simulink model "Iteration3_Transformer_classAmplifier"  (R2015a)
settings: Solver=ode23t  StartTime=0.0  StopTime=1e-2  RelTol=1e-3
libraries: fl_lib x9, elec_lib x9, nesl_utility x6
settings Model: Creator=saifur  LastModifiedBy=saifur
settings DebuggingCC: UnconnectedInputMsg=none  UnconnectedOutputMsg=none  UnconnectedLineMsg=none

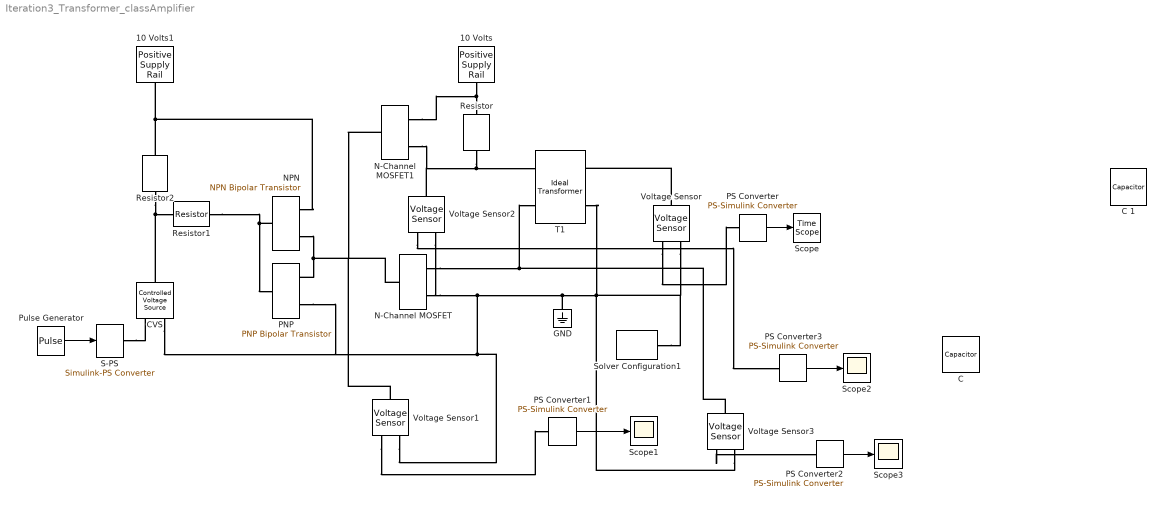
== system Iteration3_Transformer_classAmplifier ==
  " C " : fl_lib/Electrical/Electrical Elements/Capacitor  c=1e-6 F  r=1e-6 Ohm  g=0 1/Ohm  i_specify=off  i_priority=High  i=0 A  v_specify=off  v_priority=High  v=0 V  vc_specify=off  vc_priority=High  vc=0 V
  " C 1" : fl_lib/Electrical/Electrical Elements/Capacitor  c=4700e-6 F  r=1e-6 Ohm  g=0 1/Ohm  i_specify=off  i_priority=High  i=0 A  v_specify=off  v_priority=High  v=0 V  vc_specify=off  vc_priority=High  vc=0 V
  10 Volts : elec_lib/Sources/Positive Supply Rail  v0=5 V
  10 Volts1 : elec_lib/Sources/Positive Supply Rail  v0=5 V
  CVS : fl_lib/Electrical/Electrical Sources/Controlled Voltage Source
  GND : fl_lib/Electrical/Electrical Elements/Electrical Reference
  N-Channel MOSFET : elec_lib/Semiconductor Devices/N-Channel MOSFET  parameterization=1  prmDatasheet=1  prmEquCoeff=1  Beta=5 A/V^2  Rds=0.025 Ohm  Id=6 A  Vgs=10 V  Vth=1.7 V  lam=0 1/V  Tmeas=25 C  RS=1e-4 Ohm  RD=0.01 Ohm  C_param=1  C_GS=270 pF  C_GD=80 pF  C_iss=350 pF  C_rss=80 pF  C_oss=0 pF  C_GS_vec=[ 270 300 290 280 295 255 ] pF  C_GD_vec=[ 450 400 300 190 95 55 ] pF  C_iss_vec=[ 720 700 590 470 390 310 ] pF  C_rss_vec=[ 450 400 300 190 95 55 ] pF  C_oss_vec=[ 900 810 690 420 270 170 ] pF  C_Vds_vec=[ 0.1 0.3 1 3 10 30 ] V  charge_linearity_param=1  C_OX=200 pF  V_C_OX=-0.5 V  dVth_dT=-6 mV/K  Rds_T2=0.037 Ohm  Tmeas2=125 C  BEXDatasheet=-1.5  BEXEquCoeff=-1.5  TdeviceDatasheet=25 C  TdeviceEquCoeff=25 C  Rth=[ 0 10 ] K/W  thermal_mass_parameterization=1  thermal_mass=[ 0 1 ] J/K  thermal_time_constant=[ 0 10 ] s  thermal_mass_initial_temperatures=[ 25 25 ] C
  N-Channel MOSFET1 : elec_lib/Semiconductor Devices/N-Channel MOSFET  parameterization=1  prmDatasheet=1  prmEquCoeff=1  Beta=5 A/V^2  Rds=0.025 Ohm  Id=6 A  Vgs=10 V  Vth=1.7 V  lam=0 1/V  Tmeas=25 C  RS=1e-4 Ohm  RD=0.01 Ohm  C_param=1  C_GS=270 pF  C_GD=80 pF  C_iss=350 pF  C_rss=80 pF  C_oss=0 pF  C_GS_vec=[ 270 300 290 280 295 255 ] pF  C_GD_vec=[ 450 400 300 190 95 55 ] pF  C_iss_vec=[ 720 700 590 470 390 310 ] pF  C_rss_vec=[ 450 400 300 190 95 55 ] pF  C_oss_vec=[ 900 810 690 420 270 170 ] pF  C_Vds_vec=[ 0.1 0.3 1 3 10 30 ] V  charge_linearity_param=1  C_OX=200 pF  V_C_OX=-0.5 V  dVth_dT=-6 mV/K  Rds_T2=0.037 Ohm  Tmeas2=125 C  BEXDatasheet=-1.5  BEXEquCoeff=-1.5  TdeviceDatasheet=25 C  TdeviceEquCoeff=25 C  Rth=[ 0 10 ] K/W  thermal_mass_parameterization=1  thermal_mass=[ 0 1 ] J/K  thermal_time_constant=[ 0 10 ] s  thermal_mass_initial_temperatures=[ 25 25 ] C
  "NPN " : elec_lib/Semiconductor Devices/NPN Bipolar Transistor  parameterization=1  prmDatasheet=1  prmEquCoeff=1  BF=100  IS=1e-14 A  ec=1  VAF=200 V  hfe=100  hoe=5e-5 1/Ohm  Ic_h=1 mA  Vce_h=5 V  V1=0.55 V  I1=0.5 mA  BR=1  Tmeas=25 C  RC=0.01 Ohm  RE=1e-4 Ohm  RB=1 Ohm  C_BC=5 pF  C_BE=5 pF  TF=0 us  TR=0 us  hfe_T2=125  XTB=0  V1_T2=0.45 V  I1_T2=0.5 mA  Tmeas2=125 C  EG=1.11 eV  XTI=3  TdeviceDatasheet=25 C  TdeviceEquCoeff=25 C  Rth=[ 0 10 ] K/W  thermal_mass_parameterization=1  thermal_mass=[ 0 1 ] J/K  thermal_time_constant=[ 0 10 ] s  thermal_mass_initial_temperatures=[ 25 25 ] C
  "PNP " : elec_lib/Semiconductor Devices/PNP Bipolar Transistor  parameterization=1  prmDatasheet=1  prmEquCoeff=1  BF=100  IS=1e-14 A  ec=1  VAF=200 V  hfe=100  hoe=5e-5 1/Ohm  Ic_h=-1 mA  Vce_h=-5 V  V1=-0.55 V  I1=-0.5 mA  BR=1  Tmeas=25 C  RC=0.01 Ohm  RE=1e-4 Ohm  RB=1 Ohm  C_BC=5 pF  C_BE=5 pF  TF=0 us  TR=0 us  hfe_T2=125  XTB=0  V1_T2=-0.45 V  I1_T2=-0.5 mA  Tmeas2=125 C  EG=1.11 eV  XTI=3  TdeviceDatasheet=25 C  TdeviceEquCoeff=25 C  Rth=[ 0 10 ] K/W  thermal_mass_parameterization=1  thermal_mass=[ 0 1 ] J/K  thermal_time_constant=[ 0 10 ] s  thermal_mass_initial_temperatures=[ 25 25 ] C
  PS Converter{,1..3} (4 alike) : nesl_utility/PS-Simulink Converter  PhysicalDomain=network_engine_domain  SubClassName=ps_output  LeftPortType=input  RightPortType=output  PseudoPeriodic=off  Frequencies=[]  Unit=1  AffineConversion=off
  Pulse Generator : DiscretePulseGenerator  PulseType=Time based  Amplitude=5  Period=0.000005  PulseWidth=50
  Resistor : elec_lib/Passive Devices/Resistor  R=100 kOhm  noise_mode=0  Tdevice=25 C  sample_time=0.001 s  repeatability=1  auto_seed=696567710  user_seed=0
  Resistor1 : elec_lib/Passive Devices/Resistor  R=10 Ohm  noise_mode=0  Tdevice=25 C  sample_time=0.001 s  repeatability=1  auto_seed=2103192391  user_seed=0
  Resistor2 : elec_lib/Passive Devices/Resistor  R=100 Ohm  noise_mode=0  Tdevice=25 C  sample_time=0.001 s  repeatability=1  auto_seed=1458113108  user_seed=0
  "S-PS " : nesl_utility/Simulink-PS Converter  PhysicalDomain=network_engine_domain  SubClassName=ps_input  LeftPortType=input  RightPortType=output  PseudoPeriodic=off  Frequencies=[]  NoiseDistribution=none  NoiseParameters=[]  Unit=V  AffineConversion=off  InputFiltering=off  SimscapeFilterOrder=1  InputFilterTimeConstant=0.001  UdotUserProvided=1
  Scope : TimeScope
  Scope1 : Scope
      settings: YMin=1  YMax=4
  Scope2 : Scope
      settings: YMin=4.99998  YMax=4.99998  SaveName=ScopeData2
  Scope3 : Scope
      settings: YMin=-0.6  YMax=0.05  SaveName=ScopeData3
  Solver Configuration1 : nesl_utility/Solver Configuration  PhysicalDomain=network_engine_domain  SubClassName=solver  LeftPortType=input  RightPortType=generic  Accelerate=off  Tones=[]  Harmonics=[]  SimulateNoise=off  Profile=off  UseLocalSampling=off  EnableSwitchedLinearOptims=on  FrequencyDomain=off  UseCCode=off  RelTol=0.001  AbsTol=1e-06  MinStep=1e-09  ToWorkspace=off  RevertToSquareIcSolve=off  NumHomotopyIterations=100  DoDC=on  ResidualTolerance=1e-09  UseLocalSolver=off  LocalSolverChoice=NE_BACKWARD_EULER_ADVANCER  LocalSolverSampleTime=0.001  DoFixedCost=off  MaxNonlinIter=3  MaxModeIter=2  LinearAlgebra=Sparse  DelaysMemoryBudget=1024  AutomaticFiltering=on  FilteringTimeConstant=0.001
  T1 : fl_lib/Electrical/Electrical Elements/Ideal Transformer  n=0.1  i1_specify=off  i1_priority=High  i1=0 A  v1_specify=off  v1_priority=High  v1=0 V  i2_specify=off  i2_priority=High  i2=0 A  v2_specify=off  v2_priority=High  v2=0 V
  Voltage Sensor{,1..3} (4 alike) : fl_lib/Electrical/Electrical Sensors/Voltage Sensor
      settings: LogSimulationData=on
  wires:
  PS Converter/1 -> Scope/1
  Pulse Generator/1 -> "S-PS "/1
  PS Converter1/1 -> Scope1/1
  PS Converter3/1 -> Scope2/1
  PS Converter2/1 -> Scope3/1
  connections:
  Voltage Sensor/LConn1 -- T1/RConn1
  Solver Configuration1/RConn1 -- Voltage Sensor/RConn2 -- Voltage Sensor3/RConn2 -- Voltage Sensor2/RConn2 -- N-Channel MOSFET/RConn2 -- "PNP "/RConn2 -- CVS/RConn2 -- Voltage Sensor1/RConn2 -- GND/LConn1 -- T1/RConn2
  Voltage Sensor/RConn1 -- PS Converter/LConn1
  N-Channel MOSFET/RConn1 -- Voltage Sensor3/LConn1 -- T1/LConn2
  Resistor/RConn1 -- Voltage Sensor2/LConn1 -- N-Channel MOSFET1/RConn2 -- T1/LConn1
  10 Volts/RConn1 -- N-Channel MOSFET1/RConn1 -- Resistor/LConn1
  "S-PS "/RConn1 -- CVS/RConn1
  "NPN "/RConn2 -- N-Channel MOSFET1/LConn1 -- Voltage Sensor1/LConn1 -- N-Channel MOSFET/LConn1 -- "PNP "/RConn1
  "NPN "/LConn1 -- "PNP "/LConn1 -- Resistor1/LConn1
  CVS/LConn1 -- Resistor2/LConn1 -- Resistor1/RConn1
  Voltage Sensor1/RConn1 -- PS Converter1/LConn1
  Voltage Sensor2/RConn1 -- PS Converter3/LConn1
  Voltage Sensor3/RConn1 -- PS Converter2/LConn1
  Resistor2/RConn1 -- "NPN "/RConn1 -- 10 Volts1/RConn1
